simulink model "dds_test_model"  (R2022b)
settings: Solver=VariableStepDiscrete  StartTime=0.0  StopTime=sim_time  RelTol=1e-3  EnableMultiTasking=on
values from neighbouring files (symbols this model uses):
  fclk = 96    [sim_dds_test_model.m]
  L = 6    [sim_dds_test_model.m]
  Pesc = P/2^M    [sim_dds_test_model.m]
  W = 16    [sim_dds_test_model.m]
libraries: simulink x1
settings Model: Creator=jvalls  LastModifiedBy=jvc
settings SolverCC: AlgebraicLoopSolver=TrustRegion
settings DataIOCC: LimitDataPoints=on  SaveFormat=Array  ReturnWorkspaceOutputs=off
settings OptimizationCC: ReuseModelBlockBuffer=on  LifeSpan=inf
settings DebuggingCC: SolverPrmCheckMsg=warning  UnconnectedInputMsg=warning  UnconnectedOutputMsg=warning  UnconnectedLineMsg=warning  SFUnexpectedBacktrackingDiag=warning  SFNoUnconditionalDefaultTransitionDiag=warning  SFExecutionAtInitializationDiag=none  ArithmeticOperatorsInVariantConditions=warning
settings HardwareCC: ProdBitPerPointer=32  ProdBitPerSizeT=32  ProdBitPerPtrDiffT=32  ProdLargestAtomicFloat=None  ProdIntDivRoundTo=Undefined  ProdEndianess=Unspecified  ProdWordSize=32  ProdHWDeviceType=32-bit Generic
settings ModelReferenceCC: EnableRefExpFcnMdlSchedulingChecks=on  PropagateSignalLabelsOutOfModel=off
settings SFSimCC: SimUseLocalCustomCode=off  CustomCodeUndefinedFunction=UseInterfaceOnly
settings RTWCC: RTWUseLocalCustomCode=off
settings CodeAppCC: StateflowObjectComments=on
settings GRTTargetCC: TargetLangStandard=C89/C90 (ANSI)
settings ConfigComp: CovMetricSettings=dw  CovSaveCumulativeToWorkspaceVar=on  CovSaveSingleToWorkspaceVar=on  CovExternalEMLEnable=off  CovSFcnEnable=off

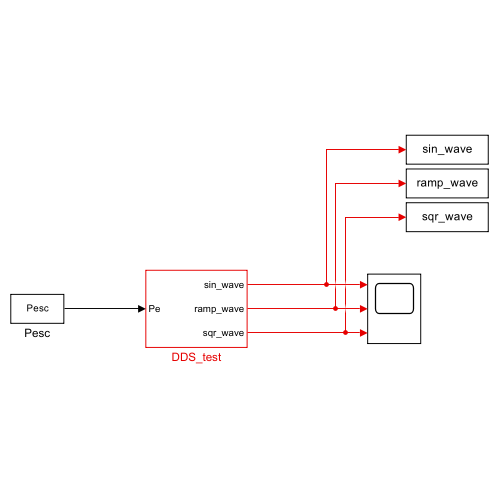
[thumbnail: Simulink's stored preview of the top-level diagram]
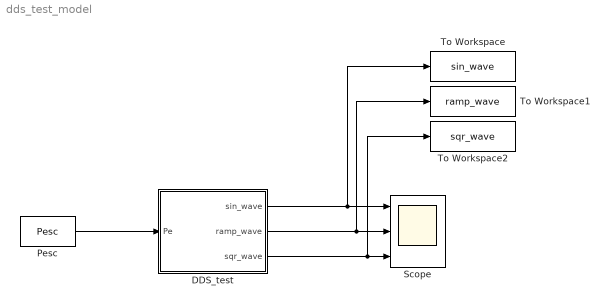
== system dds_test_model ==
  DDS_test : Subsystem
  Pesc : Constant  Value=Pesc  SampleTime=1/fclk
  Scope : Scope  NumInputPorts=3
  To Workspace : ToWorkspace  VariableName=sin_wave  SampleTime=-1
      settings: Save2DSignal=2-D array (concatenate along first dimension)
  To Workspace1 : ToWorkspace  VariableName=ramp_wave  SampleTime=-1
      settings: Save2DSignal=2-D array (concatenate along first dimension)
  To Workspace2 : ToWorkspace  VariableName=sqr_wave  SampleTime=-1
      settings: Save2DSignal=2-D array (concatenate along first dimension)
  wires:
  DDS_test/2(ramp_wave) -> To Workspace1/1, Scope/2
  DDS_test/3(sqr_wave) -> To Workspace2/1, Scope/3
  DDS_test/1(sin_wave) -> To Workspace/1, Scope/1
  Pesc/1 -> DDS_test/1(Pe)

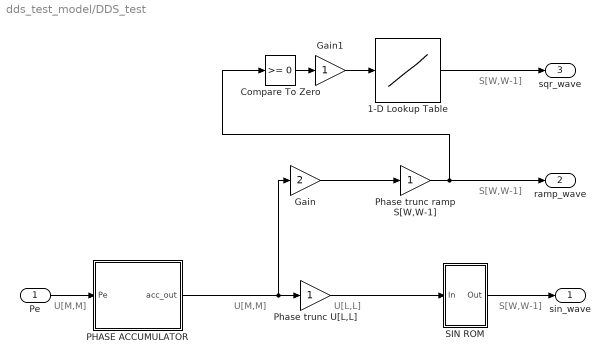
== system dds_test_model/DDS_test ==
  note: S[W,W-1]
  note: S[W,W-1]
  note: S[W,W-1]
  note: U[M,M]
  note: U[L,L]
  note: U[M,M]
  Pe : Inport
  1-D Lookup Table : Lookup_n-D  NumberOfTableDimensions=1  BreakpointsForDimension1=[0:1]  Table=[ -1+2^-(W-1) 1-2^-(W-1)]  InternalRulePriority=Speed  RndMeth=Simplest
  Compare To Zero : simulink/Logic and Bit Operations/Compare To Zero  relop=>=  OutDataTypeStr=boolean
  Gain : Gain  Gain=2
  Gain1 : Gain  OutDataTypeStr=double
  PHASE ACCUMULATOR : Subsystem
  Phase trunc U[L,L] : Gain  OutDataTypeStr=fixdt(0,L,L)
  Phase trunc ramp S[W,W-1] : Gain  OutDataTypeStr=fixdt(1,W,W-1)
  SIN ROM : Subsystem
  sin_wave : Outport  VectorParamsAs1DForOutWhenUnconnected=off
  ramp_wave : Outport  Port=2  VectorParamsAs1DForOutWhenUnconnected=off
  sqr_wave : Outport  Port=3  VectorParamsAs1DForOutWhenUnconnected=off
  wires:
  Phase trunc U[L,L]/1 -> SIN ROM/1(In)
  SIN ROM/1(Out) -> sin_wave/1
  Pe/1 -> PHASE ACCUMULATOR/1(Pe)
  Phase trunc ramp S[W,W-1]/1 -> Compare To Zero/1, ramp_wave/1
  1-D Lookup Table/1 -> sqr_wave/1
  Gain/1 -> Phase trunc ramp S[W,W-1]/1
  PHASE ACCUMULATOR/1(acc_out) -> Phase trunc U[L,L]/1, Gain/1
  Gain1/1 -> 1-D Lookup Table/1
  Compare To Zero/1 -> Gain1/1

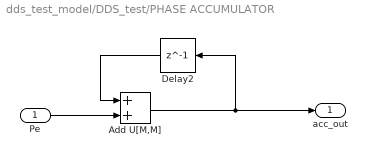
== system dds_test_model/DDS_test/PHASE ACCUMULATOR ==
  Pe : Inport
  Add U[M,M] : Sum  AccumDataTypeStr=fixdt(0,M,M)  OutDataTypeStr=fixdt(0,M,M)  RndMeth=Convergent
  Delay2 : Delay  DelayLength=1
  acc_out : Outport  VectorParamsAs1DForOutWhenUnconnected=off
  wires:
  Add U[M,M]/1 -> acc_out/1, Delay2/1
  Pe/1 -> Add U[M,M]/2
  Delay2/1 -> Add U[M,M]/1

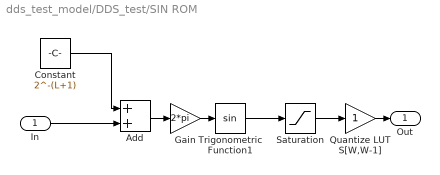
== system dds_test_model/DDS_test/SIN ROM ==
  In : Inport
  Add : Sum
  Constant : Constant  Value=2^-(L+1)
  Gain : Gain  Gain=2*pi
  Quantize LUT S[W,W-1] : Gain  OutDataTypeStr=fixdt(1,W,W-1)  RndMeth=Round  SaturateOnIntegerOverflow=on
  Saturation : Saturate  UpperLimit=1-2^-(W-1)  LowerLimit=-(1-2^-(W-1))
  Trigonometric Function1 : Trigonometry
  Out : Outport  VectorParamsAs1DForOutWhenUnconnected=off
  wires:
  Add/1 -> Gain/1
  In/1 -> Add/2
  Constant/1 -> Add/1
  Quantize LUT S[W,W-1]/1 -> Out/1
  Trigonometric Function1/1 -> Saturation/1
  Gain/1 -> Trigonometric Function1/1
  Saturation/1 -> Quantize LUT S[W,W-1]/1
